simulink model "test_Wall_in"  (R2016b)
settings: Solver=ode23tb  StartTime=0.0  StopTime=100*24*3600  RelTol=1e-3  EnableMultiTasking=on
libraries: carnot x6
settings Model: Creator=drhf  LastModifiedBy=drhf
settings DataIOCC: LimitDataPoints=on  SaveFormat=Array  SignalLoggingSaveFormat=ModelDataLogs
settings OptimizationCC: ExpressionDepthLimit=2147483647  LifeSpan=inf
settings DebuggingCC: UnderspecifiedInitializationDetection=Classic  MergeDetectMultiDrivingBlocksExec=none  SolverPrmCheckMsg=warning  StateNameClashWarn=warning  SFUnexpectedBacktrackingDiag=warning  SFNoUnconditionalDefaultTransitionDiag=warning  SFExecutionAtInitializationDiag=none
settings HardwareCC: ProdBitPerPointer=32  ProdBitPerSizeT=32  ProdBitPerPtrDiffT=32  ProdLargestAtomicFloat=None  ProdIntDivRoundTo=Undefined  ProdEndianess=Unspecified  ProdWordSize=32  ProdHWDeviceType=32-bit Generic
settings ModelReferenceCC: PropagateSignalLabelsOutOfModel=off
settings GRTTargetCC: TargetLangStandard=C89/C90 (ANSI)  GeneratePreprocessorConditionals=Disable all  CombineOutputUpdateFcns=off  GRTInterface=on
settings ConfigComp: CovMetricSettings=dw  CovHtmlReporting=on  CovSaveCumulativeToWorkspaceVar=on  CovSaveSingleToWorkspaceVar=on  CovExternalEMLEnable=off

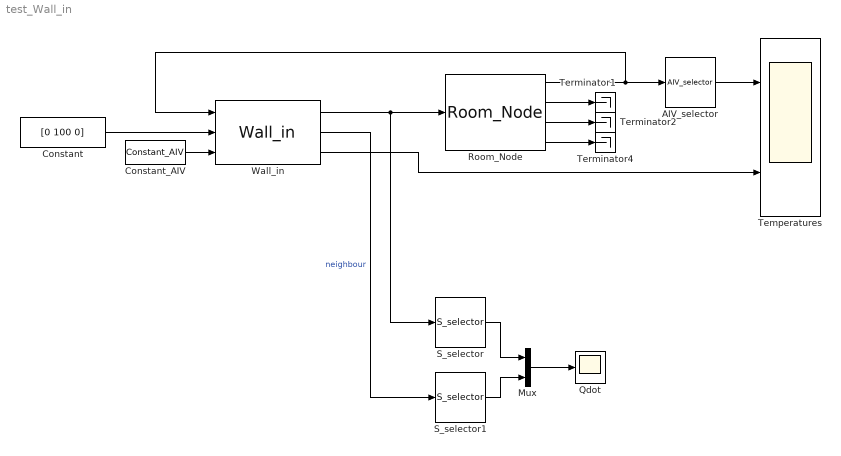
== system test_Wall_in ==
  AIV_selector : carnot/Outputs/AIV_selector  e1=on  e2=off  e3=off  e4=off  e5=off  e6=off  e7=off  e8=off  e9=off
  Constant : Constant  Value=[0 100 0]
  Constant_AIV : carnot/Source/Ventilation/Constant_AIV  Tsens=20  Tcon=20  Trad=20  mw=0.012  mco=0.01  rhoair=1.2  cpair=1004  pair=100000  nair=0.5
  Mux : Mux  Inputs=2
  Qdot : Scope
  Room_Node : carnot/Load/Houses/room_nodes/Room_Node  zoneairvolume=5*5*2.5  zoneheight=2.5  zonestartTEMP=20  zonestartWATER=55  timeconst=100  heatperfect=natural  lookuptime=[0 24]*3600  lookupvalue=[20 20]  AirPressure=101300
  S_selector : carnot/Outputs/S_selector  e1=off  e2=off  e3=off  e4=off  e5=on  e6=off  e7=off  e8=off  e9=off  e10=off  e11=off  e12=off  e13=off
  S_selector1 : carnot/Outputs/S_selector  e1=off  e2=off  e3=off  e4=off  e5=on  e6=off  e7=off  e8=off  e9=off  e10=off  e11=off  e12=off  e13=off
  Temperatures : Scope  NumInputPorts=2
  Terminator1 : Terminator
  Terminator2 : Terminator
  Terminator4 : Terminator
  Wall_in : carnot/Load/Houses/wall_floor/Wall_in  wallsize=[10 10]  d=[0.1 0.1 0.1]  cond=[1 1 1]  cwall=[0.28 0.28 0.28]*3600  rho=[2000 200 2000]  emission_in=.96  dactive=[0.05 0.15 0.25]  t0=20  tau=1000*3600
  wires:
  Wall_in/1 -> S_selector/1, Room_Node/1
  Wall_in/2 -> S_selector1/1  "neighbour"
  Room_Node/1 -> AIV_selector/1, Wall_in/1
  Constant/1 -> Wall_in/2
  AIV_selector/1 -> Temperatures/1
  Mux/1 -> Qdot/1
  S_selector/1 -> Mux/1
  S_selector1/1 -> Mux/2
  Room_Node/2 -> Terminator1/1
  Room_Node/3 -> Terminator2/1
  Wall_in/3 -> Temperatures/2
  Room_Node/4 -> Terminator4/1
  Constant_AIV/1 -> Wall_in/3
